simulink model "RBFNNfaultdet"  (R2020b)
settings: Solver=ode23tb  StartTime=0.0  StopTime=0.15  RelTol=1e-3  EnableMultiTasking=on
libraries: powerlib x13
settings Model: Creator=Rodney Tan  LastModifiedBy=Prabin
settings DataIOCC: LimitDataPoints=on  SaveFormat=Array  ReturnWorkspaceOutputs=off
settings OptimizationCC: LifeSpan=inf
settings DebuggingCC: SFUnexpectedBacktrackingDiag=warning  SFNoUnconditionalDefaultTransitionDiag=warning  SFExecutionAtInitializationDiag=none  ArithmeticOperatorsInVariantConditions=warning
settings HardwareCC: ProdBitPerPointer=32  ProdBitPerSizeT=32  ProdBitPerPtrDiffT=32  ProdLargestAtomicFloat=None  ProdIntDivRoundTo=Undefined  ProdEndianess=Unspecified  ProdWordSize=32  ProdHWDeviceType=32-bit Generic
settings ModelReferenceCC: PropagateSignalLabelsOutOfModel=off
settings SFSimCC: SimUseLocalCustomCode=off  CustomCodeUndefinedFunction=UseInterfaceOnly
settings RTWCC: RTWUseLocalCustomCode=off
settings CodeAppCC: StateflowObjectComments=on
settings GRTTargetCC: TargetLangStandard=C89/C90 (ANSI)
settings ConfigComp: CovMetricSettings=dw  CovSaveCumulativeToWorkspaceVar=on  CovSaveSingleToWorkspaceVar=on  CovExternalEMLEnable=off
settings SimscapeCC: SimscapeNormalizeSystem=off

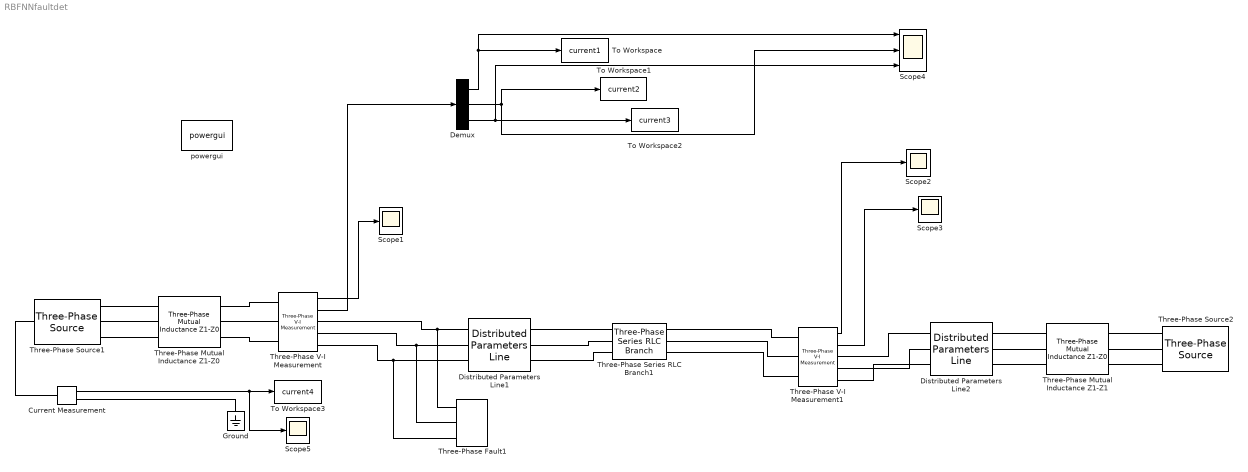
== system RBFNNfaultdet ==
  Current Measurement : powerlib/Measurements/Current Measurement  PhasorSimulation=off  OutputType=Complex  PSBequivalent=0
  Demux : Demux  Outputs=3
  Distributed Parameters Line1 : powerlib/Elements/Distributed Parameters Line  Phases=3  Length=100  Frequency=50  Resistance=[2.34/100 38.85/100]  Inductance="[95.10e-3/100  325.08e-3/100]"  Capacitance=[1.24e-6/100 .845e-6/100]  x1=[1.77628762550502e-10 400715.111368201 400715.111368201;314.159265358979 314.159265358979 314.159265358979;2.01686788663 0.415584579860558 -1.15521174693434]  x2=[7.83644617642058e-11 402600.717466212 402600.717466212;314.159265358979 314.159265358979 314.159265358979;2.59643187192332 0.415379454862749 -1.15541687193215]  x3=[1.72900381756988e-12 1446.8094117599 1446.80941175991;314.159265358979 314.159265358979 314.159265358979;-2.91390691392838 0.318253399265251 -1.25254292752965]  x4=[1.39478366240956e-12 1442.49876820066 1442.49876820066;314.159265358979 314.159265358979 314.159265358979;2.81828298684929 0.404728643975136 -1.16606768281976]  x5=0.000524111247732769  V1=[1.776e-10 4.007e+05 4.007e+05;314.2 314.2 314.2;2.017 0.4156 -1.155]  V2=[7.836e-11 4.026e+05 4.026e+05;314.2 314.2 314.2;2.596 0.4154 -1.155]  I1=[1.729e-12 1447 1447;314.2 314.2 314.2;-2.914 0.3183 -1.253]  I2=[1.395e-12 1442 1442;314.2 314.2 314.2;2.818 0.4047 -1.166]  nHarmo=1  Measurements=None  Decoupling=off  VsMag0=0  VrMag0=0  VsAngle0=0  VrAngle0=0  IsMag0=0  IrMag0=0  IsAngle0=0  IrAngle0=0
  Distributed Parameters Line2 : powerlib/Elements/Distributed Parameters Line  Phases=3  Length=100  Frequency=50  Resistance=[2.34/100 38.85/100]  Inductance="[95.10e-3/100  325.08e-3/100]"  Capacitance=[1.24e-6/100 .845e-6/100]  x1=[6.21658091063548e-10 407268.099951264 407268.099951265;314.159265358979 314.159265358979 314.159265358979;1.89233926769478 0.360051012902 -1.2107453138929]  x2=[6.50781433068853e-11 401266.456613997 401266.456613997;314.159265358979 314.159265358979 314.159265358979;0.860167110962933 0.36146100387797 -1.20933532291693]  x3=[2.20767850305269e-12 1458.94116184067 1458.94116184067;314.159265358979 314.159265358979 314.159265358979;-2.30340002692352 0.370561610595407 -1.20023471619949]  x4=[4.67926624546127e-12 1454.60110788861 1454.60110788861;314.159265358979 314.159265358979 314.159265358979;0.554808530874296 0.188330115256826 -1.38246621153807]  x5=0.000786166871599153  V1=[6.217e-10 4.073e+05 4.073e+05;314.2 314.2 314.2;1.892 0.3601 -1.211]  V2=[6.508e-11 4.013e+05 4.013e+05;314.2 314.2 314.2;0.8602 0.3615 -1.209]  I1=[2.208e-12 1459 1459;314.2 314.2 314.2;-2.303 0.3706 -1.2]  I2=[4.679e-12 1455 1455;314.2 314.2 314.2;0.5548 0.1883 -1.382]  nHarmo=1  Measurements=None  Decoupling=off  VsMag0=0  VrMag0=0  VsAngle0=0  VrAngle0=0  IsMag0=0  IrMag0=0  IsAngle0=0  IrAngle0=0
  Ground : powerlib/Elements/Ground  LConnTagsString=a
  Scope{1..3,5} (4 alike) : Scope
  Scope4 : Scope  NumInputPorts=3
  Three-Phase Mutual Inductance Z1-Z0 : powerlib/Elements/Three-Phase Mutual Inductance Z1-Z0  LConnTagsString=a|b|c  RConnTagsString=A|B|C  PositiveSequence="[ 0.45  0.016]"  ZeroSequence=[0.675 0.024]
      settings: SourceProductBaseCode=PS
  Three-Phase Mutual Inductance Z1-Z1 : powerlib/Elements/Three-Phase Mutual Inductance Z1-Z0  LConnTagsString=a|b|c  RConnTagsString=A|B|C  PositiveSequence="[ 0.45  0.016]"  ZeroSequence=[0.675 0.024]
      settings: SourceProductBaseCode=PS
  Three-Phase Series RLC Branch1 : powerlib/Elements/Three-Phase Series RLC Branch  LConnTagsString=A|B|C  RConnTagsString=A|B|C  BranchType=RLC  Resistance=6  Inductance=0.053052  Capacitance=1e-5  Measurements=None
  Three-Phase V-I Measurement : powerlib/Measurements/Three-Phase V-I Measurement  VoltageMeasurement=phase-to-ground  SetLabelV=off  LabelV=Vabc  Vpu=on  VpuLL=off  CurrentMeasurement=yes  SetLabelI=off  LabelI=Iabc  Ipu=on  Pbase=500e6  Vbase=400e3  OutputType=Complex  PhasorSimulation=off  PSBequivalent=0
  Three-Phase V-I Measurement1 : powerlib/Measurements/Three-Phase V-I Measurement  VoltageMeasurement=phase-to-ground  SetLabelV=off  LabelV=Vabc  Vpu=on  VpuLL=off  CurrentMeasurement=yes  SetLabelI=off  LabelI=Iabc  Ipu=on  Pbase=400e6  Vbase=500e3  OutputType=Complex  PhasorSimulation=off  PSBequivalent=0
  Three-Phase Fault1 : powerlib/Elements/Three-Phase Fault  InitialStates=0  FaultA=on  FaultB=on  FaultC=off  GroundFault=off  SwitchTimes=[0.02]  External=off  SwitchStatus=NaN  FaultResistance=0.001  GroundResistance=0.01  SnubberResistance=1e6  SnubberCapacitance=inf  Measurements=None
  Three-Phase Source1 : powerlib/Electrical Sources/Three-Phase Source  InternalConnection=Yn  VoltagePhases=off  Voltage=400e3  PhaseAngle=0  Voltage_phases=[25e3 25e3 25e3]/sqrt(3)  PhaseAngles_phases=[0 -120 +120]  Frequency=50  NonIdealSource=on  SpecifyImpedance=off  Resistance=0.0001  Inductance=0.0001  ShortCircuitLevel=100e6  BaseVoltage=400e3  XRratio=7  BusType=swing  Pref=10e3  Qref=0  Prefabc=[10e3, 10e3, 10e3]  Qrefabc=[0, 0, 0]  Qmin=-inf  Qmax=inf
  Three-Phase Source2 : powerlib/Electrical Sources/Three-Phase Source  InternalConnection=Yg  VoltagePhases=off  Voltage=400e3  PhaseAngle=0  Voltage_phases=[25e3 25e3 25e3]/sqrt(3)  PhaseAngles_phases=[0 -120 +120]  Frequency=50  NonIdealSource=on  SpecifyImpedance=off  Resistance=.0001  Inductance=0  ShortCircuitLevel=500e6  BaseVoltage=400e3  XRratio=7  BusType=swing  Pref=10e3  Qref=0  Prefabc=[10e3, 10e3, 10e3]  Qrefabc=[0, 0, 0]  Qmin=-inf  Qmax=inf
  To Workspace : ToWorkspace  VariableName=current1  SampleTime=-1
  To Workspace1 : ToWorkspace  VariableName=current2  SampleTime=-1
  To Workspace2 : ToWorkspace  VariableName=current3  SampleTime=-1
  To Workspace3 : ToWorkspace  VariableName=current4  SampleTime=-1
  powergui : powerlib/powergui  Priority=1  SimulationMode=Continuous  SampleTime=50e-6  frequency=60  Iterations=50  frequencyindice=50  Pbase=100e6  ErrMax=1e-4  UnitsV=kV  UnitsW=MW  buscounter=0  FunctionMessages=off  echomessages=off  EnableUseOfTLC=off  CurrentSourceSwitches=off  DisableSnubberDevices=on  DisableRonSwitches=off  DisableVfSwitches=off  DisplayEquations=off  AutomaticDiscreteSolvers=off  SolverType=Tustin/Backward Euler (TBE)  Interpol=off  ExternalGateDelay=off  methode=off  Ts=100  x0status=blocks  SPID=on  SwTol=0  HookPort=off  NonlinearTolerance=1e-4  nMaxIteration=100  ContinueOnMaxIteration=off  RestoreLinks=warning  ResistiveCurrentMeasurement=off  Frange=[0:2:500]  Ylog=off  Xlog=on  ShowGrid=off  save=off  variable=ZData  structure=0  ZoomFFT=off  StartTime=0.0  cycles=1  DisplayStyle=1  fundamental=60  FreqAxis=off  MaxFrequency=1000  frequencyindicesteady=1  RmsSteady=1  display=off
  wires:
  Three-Phase V-I Measurement/1 -> Scope1/1
  Three-Phase V-I Measurement1/1 -> Scope2/1
  Three-Phase V-I Measurement1/2 -> Scope3/1
  Three-Phase V-I Measurement/2 -> Demux/1
  Demux/1 -> Scope4/1, To Workspace/1
  Demux/2 -> Scope4/2, To Workspace1/1
  Demux/3 -> To Workspace2/1, Scope4/3
  Current Measurement/1 -> Scope5/1, To Workspace3/1
  connections:
  Distributed Parameters Line1/LConn2 -- Three-Phase Fault1/LConn2 -- Three-Phase V-I Measurement/RConn2
  Distributed Parameters Line1/LConn1 -- Three-Phase Fault1/LConn1 -- Three-Phase V-I Measurement/RConn1
  Distributed Parameters Line1/LConn3 -- Three-Phase Fault1/LConn3 -- Three-Phase V-I Measurement/RConn3
  Three-Phase Series RLC Branch1/RConn1 -- Three-Phase V-I Measurement1/LConn1
  Three-Phase V-I Measurement1/LConn3 -- Three-Phase Series RLC Branch1/RConn3
  Three-Phase Series RLC Branch1/RConn2 -- Three-Phase V-I Measurement1/LConn2
  Ground/LConn1 -- Current Measurement/RConn1
  Distributed Parameters Line1/RConn3 -- Three-Phase Series RLC Branch1/LConn3
  Distributed Parameters Line1/RConn2 -- Three-Phase Series RLC Branch1/LConn2
  Distributed Parameters Line1/RConn1 -- Three-Phase Series RLC Branch1/LConn1
  Three-Phase Mutual Inductance Z1-Z1/RConn1 -- Three-Phase Source2/RConn1
  Three-Phase Mutual Inductance Z1-Z1/RConn2 -- Three-Phase Source2/RConn2
  Three-Phase Mutual Inductance Z1-Z1/RConn3 -- Three-Phase Source2/RConn3
  Three-Phase V-I Measurement1/RConn1 -- Distributed Parameters Line2/LConn1
  Three-Phase V-I Measurement1/RConn2 -- Distributed Parameters Line2/LConn2
  Three-Phase V-I Measurement1/RConn3 -- Distributed Parameters Line2/LConn3
  Distributed Parameters Line2/RConn1 -- Three-Phase Mutual Inductance Z1-Z1/LConn1
  Distributed Parameters Line2/RConn2 -- Three-Phase Mutual Inductance Z1-Z1/LConn2
  Distributed Parameters Line2/RConn3 -- Three-Phase Mutual Inductance Z1-Z1/LConn3
  Three-Phase Mutual Inductance Z1-Z0/LConn1 -- Three-Phase Source1/RConn1
  Three-Phase Mutual Inductance Z1-Z0/LConn2 -- Three-Phase Source1/RConn2
  Three-Phase Mutual Inductance Z1-Z0/LConn3 -- Three-Phase Source1/RConn3
  Three-Phase Mutual Inductance Z1-Z0/RConn1 -- Three-Phase V-I Measurement/LConn1
  Three-Phase Mutual Inductance Z1-Z0/RConn2 -- Three-Phase V-I Measurement/LConn2
  Three-Phase Mutual Inductance Z1-Z0/RConn3 -- Three-Phase V-I Measurement/LConn3
  Three-Phase Source1/LConn1 -- Current Measurement/LConn1
